simulink model "simulink_benchmark"  (R2023b)
settings: Solver=ode45  StartTime=0  StopTime=39.7995  RelTol=1e-3
undefined symbols (not defined in the file or in its folder): tau_s
settings Model: Creator=Previ  LastModifiedBy=Previ

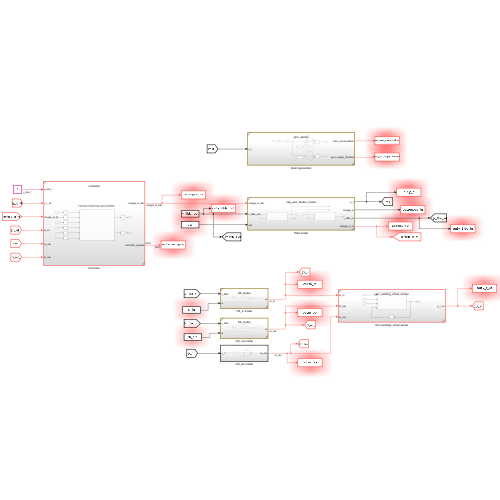
[thumbnail: Simulink's stored preview of the top-level diagram]
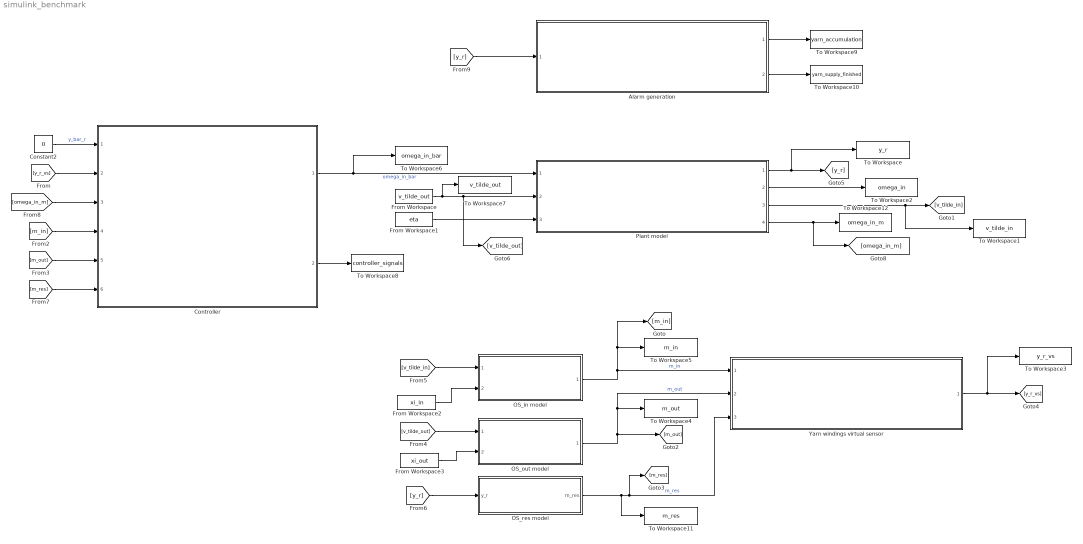
== system simulink_benchmark ==
  Alarm generation : Subsystem  ReferencedSubsystem=yarn_alarms
  Constant2 : Constant  Value=0
  Controller : Subsystem  ReferencedSubsystem=controller
  From Workspace : FromWorkspace  VariableName=v_tilde_out
  From Workspace1 : FromWorkspace  VariableName=eta
  From Workspace2 : FromWorkspace  VariableName=xi_in
  From Workspace3 : FromWorkspace  VariableName=xi_out
  OS_in model : Subsystem  ReferencedSubsystem=OS_model
  OS_out model : Subsystem  ReferencedSubsystem=OS_model
  OS_res model : Subsystem
  Plant model : Subsystem  ReferencedSubsystem=neg_yarn_feeder_model
  To Workspace : ToWorkspace  VariableName=y_r  SaveFormat=Timeseries  SampleTime=tau_s
  To Workspace1 : ToWorkspace  VariableName=v_tilde_in  SaveFormat=Timeseries  SampleTime=tau_s
  To Workspace10 : ToWorkspace  VariableName=yarn_supply_finished  SaveFormat=Timeseries  SampleTime=tau_s
  To Workspace11 : ToWorkspace  VariableName=m_res  SaveFormat=Timeseries  SampleTime=tau_s
  To Workspace12 : ToWorkspace  VariableName=omega_in_m  SaveFormat=Timeseries  SampleTime=tau_s
  To Workspace2 : ToWorkspace  VariableName=omega_in  SaveFormat=Timeseries  SampleTime=tau_s
  To Workspace3 : ToWorkspace  VariableName=y_r_vs  SaveFormat=Timeseries  SampleTime=tau_s
  To Workspace4 : ToWorkspace  VariableName=m_out  SaveFormat=Timeseries  SampleTime=tau_s
  To Workspace5 : ToWorkspace  VariableName=m_in  SaveFormat=Timeseries  SampleTime=tau_s
  To Workspace6 : ToWorkspace  VariableName=omega_in_bar  SaveFormat=Timeseries  SampleTime=tau_s
  To Workspace7 : ToWorkspace  VariableName=v_tilde_out  SaveFormat=Timeseries  SampleTime=tau_s
  To Workspace8 : ToWorkspace  VariableName=controller_signals  SaveFormat=Timeseries  SampleTime=tau_s
  To Workspace9 : ToWorkspace  VariableName=yarn_accumulation  SaveFormat=Timeseries  SampleTime=tau_s
  Yarn windings virtual sensor : Subsystem  ReferencedSubsystem=yarn_winding_virtual_sensor
  wires:
  Controller/1 -> Plant model/1, To Workspace6/1  "omega_in_bar"
  From Workspace1/1 -> Plant model/3
  From Workspace/1 -> To Workspace7/1, [v_tilde_out], Plant model/2
  Plant model/3 -> To Workspace1/1, [v_tilde_in]
  Yarn windings virtual sensor/1 -> To Workspace3/1, [y_r_vs]
  Plant model/2 -> To Workspace2/1
  [y_r] -> Alarm generation/1
  Alarm generation/1 -> To Workspace9/1
  Alarm generation/2 -> To Workspace10/1
  Constant2/1 -> Controller/1  "y_bar_r"
  [y_r_vs] -> Controller/2
  [omega_in_m] -> Controller/3
  [m_in] -> Controller/4
  [m_out] -> Controller/5
  Controller/2 -> To Workspace8/1
  Plant model/1 -> [y_r], To Workspace/1
  [v_tilde_in] -> OS_in model/1
  [v_tilde_out] -> OS_out model/1
  OS_in model/1 -> Yarn windings virtual sensor/1, [m_in], To Workspace5/1  "m_in"
  OS_out model/1 -> [m_out], To Workspace4/1, Yarn windings virtual sensor/2  "m_out"
  [y_r] -> OS_res model/1(y_r)
  OS_res model/1(m_res) -> To Workspace11/1, [m_res], Yarn windings virtual sensor/3  "m_res"
  [m_res] -> Controller/6
  Plant model/4 -> [omega_in_m], To Workspace12/1
  From Workspace2/1 -> OS_in model/2
  From Workspace3/1 -> OS_out model/2

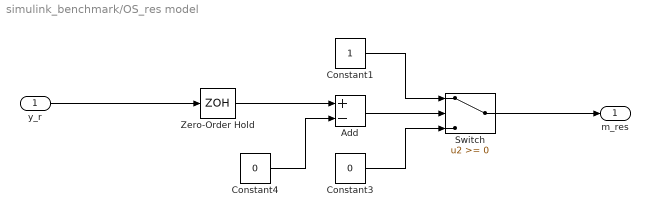
== system simulink_benchmark/OS_res model ==
  y_r : Inport
  Add : Sum  Inputs=+-
  Constant1 : Constant
  Constant3 : Constant  Value=0
  Constant4 : Constant  Value=0
  Switch : Switch  SaturateOnIntegerOverflow=off  InputSameDT=off
  Zero-Order Hold : ZeroOrderHold  SampleTime=tau_s
  m_res : Outport
  wires:
  Constant4/1 -> Add/2
  Constant3/1 -> Switch/3
  Add/1 -> Switch/2
  y_r/1 -> Zero-Order Hold/1
  Constant1/1 -> Switch/1
  Zero-Order Hold/1 -> Add/1
  Switch/1 -> m_res/1
